simulink library "symbols"  (Simulink 7.5)
settings: Solver=ode45  StartTime=0.0  StopTime=10.0  RelTol=1e-3
libraries: xbsIndex_r4 x41
settings Model: Creator=ich  LastModifiedBy=ich

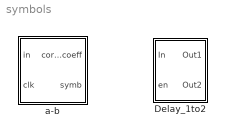
== system symbols ==
  Delay_1to2 : Subsystem
      mask Display:
      | disp('z^{-1}','texmode','on')
      | port_label('input',1,'in')
      | port_label('input',2,'en')
      | port_label('output',1,'out')
      | port_label('output',2,'out')
  a-b : Subsystem  mask{a=0, b=8, chip_a=1618456172}
      mask prompts: a "Symbol a"; b "Symbol b"; chip_a "Chipping seq. for a"

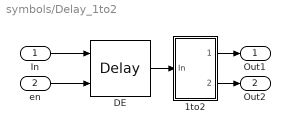
== system symbols/Delay_1to2 ==
  In : Inport
  en : Inport  Port=2
  1to2 : Subsystem
  DE : xbsIndex_r4/Delay  en=on  latency=1  dbl_ovrd=off  reg_retiming=off  block_type=delay
      settings: xl_area=[1 1 0 0 0 0 0]  block_version=12.1
  Out1 : Outport
  Out2 : Outport  Port=2
  wires:
  DE/1 -> 1to2/1(In)
  In/1 -> DE/1
  1to2/1(Out1) -> Out1/1
  1to2/2(Out2) -> Out2/1
  en/1 -> DE/2

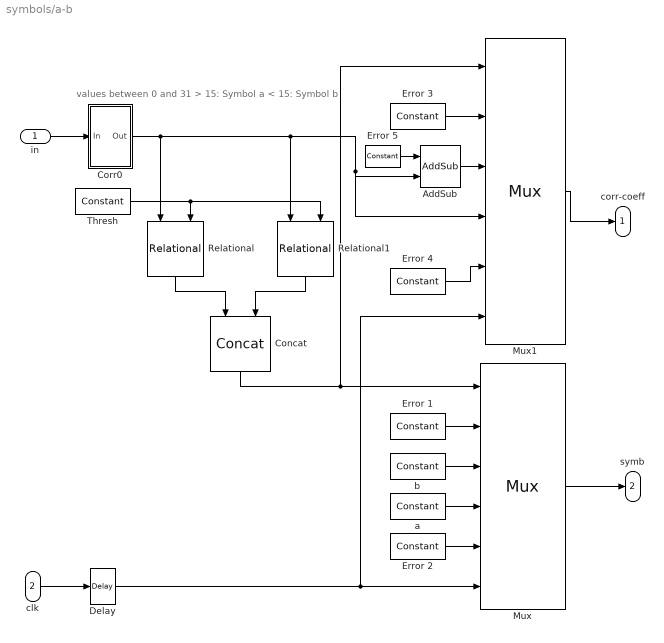
== system symbols/a-b ==
  note: values between 0 and 31
      | > 15: Symbol a
      | < 15: Symbol b
  in : Inport
  clk : Inport  Port=2
  AddSub : xbsIndex_r4/AddSub  mode=Subtraction  use_carryin=off  use_carryout=off  en=off  latency=0  precision=Full  arith_type=Unsigned  n_bits=16  bin_pt=14  quantization=Truncate  overflow=Wrap  dbl_ovrd=off  use_behavioral_HDL=off  hw_selection=Fabric  pipelined=off  block_type=addsub
      settings: block_version=12.2
  Concat : xbsIndex_r4/Concat  num_inputs=2  dbl_ovrd=off  block_type=concat
      settings: block_version=12.1
  Corr0 : Subsystem
  Delay : xbsIndex_r4/Delay  en=off  latency=1  dbl_ovrd=off  reg_retiming=off  block_type=delay
      settings: block_version=12.2
  Error 1 : xbsIndex_r4/Constant  arith_type=Unsigned  const=16  n_bits=5  bin_pt=0  explicit_period=off  period=1  equ=P=C  opselect=C  inp2=PCIN>>17  opr=+  inp1=P  carry=CIN  dbl_ovrd=off  block_type=constant
      settings: block_version=12.1
  Error 2 : xbsIndex_r4/Constant  arith_type=Unsigned  const=16  n_bits=5  bin_pt=0  explicit_period=off  period=1  equ=P=C  opselect=C  inp2=PCIN>>17  opr=+  inp1=P  carry=CIN  dbl_ovrd=off  block_type=constant
      settings: block_version=12.1
  Error 3 : xbsIndex_r4/Constant  arith_type=Unsigned  const=0  n_bits=5  bin_pt=0  explicit_period=off  period=1  equ=P=C  opselect=C  inp2=PCIN>>17  opr=+  inp1=P  carry=CIN  dbl_ovrd=off  block_type=constant
      settings: block_version=12.1
  Error 4 : xbsIndex_r4/Constant  arith_type=Unsigned  const=0  n_bits=5  bin_pt=0  explicit_period=off  period=1  equ=P=C  opselect=C  inp2=PCIN>>17  opr=+  inp1=P  carry=CIN  dbl_ovrd=off  block_type=constant
      settings: block_version=12.1
  Error 5 : xbsIndex_r4/Constant  arith_type=Unsigned  const=31  n_bits=5  bin_pt=0  explicit_period=off  period=1  equ=P=C  opselect=C  inp2=PCIN>>17  opr=+  inp1=P  carry=CIN  dbl_ovrd=off  block_type=constant
      settings: block_version=12.1
  Mux : xbsIndex_r4/Mux  inputs=4  en=on  latency=1  precision=Full  arith_type=Unsigned  n_bits=16  bin_pt=14  quantization=Truncate  overflow=Wrap  dbl_ovrd=off  block_type=mux
      settings: xl_area=[5 5 0 10 0 0 0]  block_version=12.1
  Mux1 : xbsIndex_r4/Mux  inputs=4  en=on  latency=1  precision=Full  arith_type=Unsigned  n_bits=16  bin_pt=14  quantization=Truncate  overflow=Wrap  dbl_ovrd=off  block_type=mux
      settings: xl_area=[5 5 0 10 0 0 0]  block_version=12.1
  Relational : xbsIndex_r4/Relational  mode=a>b  en=off  latency=0  dbl_ovrd=off  block_type=relational
      settings: xl_area=[4 1 0 7 0 0 0]  block_version=12.1
  Relational1 : xbsIndex_r4/Relational  mode=a<=b  en=off  latency=0  dbl_ovrd=off  block_type=relational
      settings: xl_area=[4 1 0 7 0 0 0]  block_version=12.1
  Thresh : xbsIndex_r4/Constant  arith_type=Unsigned  const=15  n_bits=5  bin_pt=0  explicit_period=off  period=1  equ=P=C  opselect=C  inp2=PCIN>>17  opr=+  inp1=P  carry=CIN  dbl_ovrd=off  block_type=constant
      settings: block_version=12.1
  a : xbsIndex_r4/Constant  arith_type=Unsigned  const=a  n_bits=5  bin_pt=0  explicit_period=off  period=1  equ=P=C  opselect=C  inp2=PCIN>>17  opr=+  inp1=P  carry=CIN  dbl_ovrd=off  block_type=constant
      settings: block_version=12.1
  b : xbsIndex_r4/Constant  arith_type=Unsigned  const=b  n_bits=5  bin_pt=0  explicit_period=off  period=1  equ=P=C  opselect=C  inp2=PCIN>>17  opr=+  inp1=P  carry=CIN  dbl_ovrd=off  block_type=constant
      settings: block_version=12.1
  corr-coeff : Outport
  symb : Outport  Port=2
  wires:
  Corr0/1(Out) -> Relational/1, Relational1/1, Mux1/4, AddSub/2
  Thresh/1 -> Relational/2, Relational1/2
  in/1 -> Corr0/1(In)
  Relational/1 -> Concat/1
  Relational1/1 -> Concat/2
  Error 1/1 -> Mux/2
  b/1 -> Mux/3
  a/1 -> Mux/4
  Error 2/1 -> Mux/5
  clk/1 -> Delay/1
  Concat/1 -> Mux/1, Mux1/1
  Mux/1 -> symb/1
  Error 3/1 -> Mux1/2
  Error 4/1 -> Mux1/5
  Mux1/1 -> corr-coeff/1
  AddSub/1 -> Mux1/3
  Error 5/1 -> AddSub/1
  Delay/1 -> Mux/6, Mux1/6

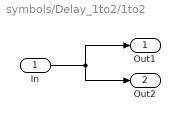
== system symbols/Delay_1to2/1to2 ==
  In : Inport  OutDataType=fixdt(1, 16)  OutScaling=2^0
  Out1 : Outport  OutDataType=fixdt(1, 16)  OutScaling=2^0
  Out2 : Outport  Port=2  OutDataType=fixdt(1, 16)  OutScaling=2^0
  wires:
  In/1 -> Out1/1, Out2/1

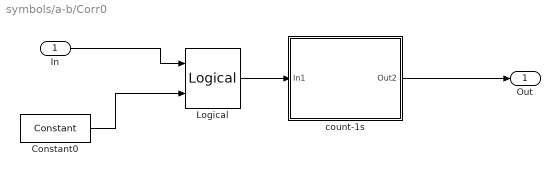
== system symbols/a-b/Corr0 ==
  In : Inport
  Constant0 : xbsIndex_r4/Constant  arith_type=Unsigned  const=chip_a  n_bits=31  bin_pt=0  explicit_period=off  period=1/8  equ=P=C  opselect=C  inp2=PCIN>>17  opr=+  inp1=P  carry=CIN  dbl_ovrd=off  block_type=constant
      settings: block_version=12.1
  Logical : xbsIndex_r4/Logical  logical_function=XNOR  inputs=2  en=off  latency=0  precision=User Defined  arith_type=Unsigned  n_bits=32  bin_pt=0  align_bp=on  dbl_ovrd=off  block_type=logical
      settings: xl_area=[31 0 0 31 0 0 0]  block_version=12.1
  count-1s : Subsystem
  Out : Outport
  wires:
  Constant0/1 -> Logical/2
  Logical/1 -> count-1s/1(In1)
  In/1 -> Logical/1
  count-1s/1(Out2) -> Out/1

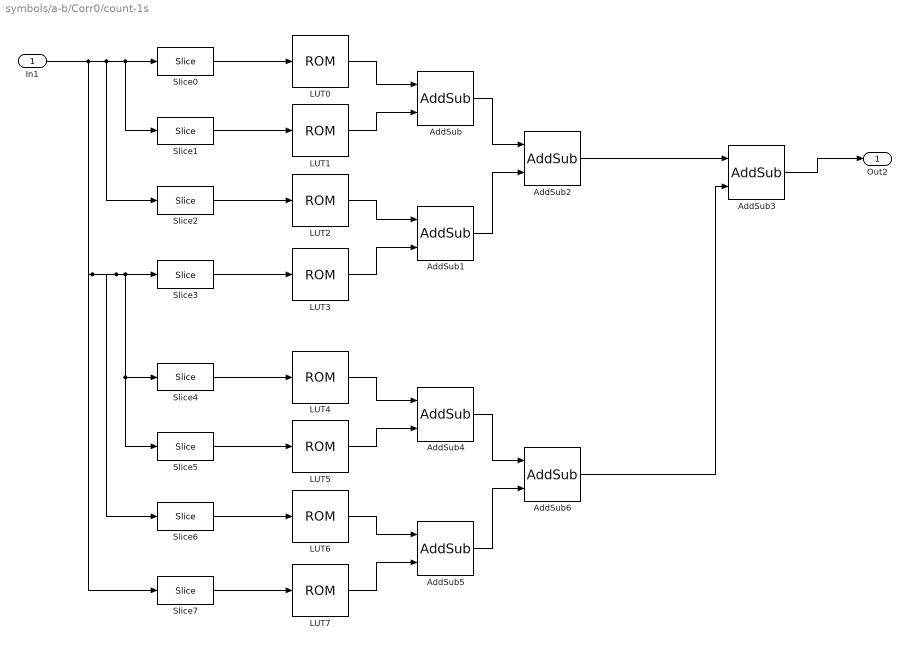
== system symbols/a-b/Corr0/count-1s ==
  In1 : Inport
  AddSub{,1,4..5} (4 alike) : xbsIndex_r4/AddSub  mode=Addition  use_carryin=off  use_carryout=off  en=off  latency=1  precision=Full  arith_type=Unsigned  n_bits=16  bin_pt=14  quantization=Truncate  overflow=Wrap  dbl_ovrd=off  use_behavioral_HDL=off  hw_selection=Fabric  pipelined=off  block_type=addsub
      settings: xl_area=[2 0 0 3 0 0 0]  block_version=12.1
  AddSub2 : xbsIndex_r4/AddSub  mode=Addition  use_carryin=off  use_carryout=off  en=off  latency=0  precision=Full  arith_type=Unsigned  n_bits=16  bin_pt=14  quantization=Truncate  overflow=Wrap  dbl_ovrd=off  use_behavioral_HDL=off  hw_selection=Fabric  pipelined=off  block_type=addsub
      settings: xl_area=[3 0 0 4 0 0 0]  block_version=12.1
  AddSub3 : xbsIndex_r4/AddSub  mode=Addition  use_carryin=off  use_carryout=off  en=off  latency=0  precision=Full  arith_type=Unsigned  n_bits=16  bin_pt=14  quantization=Truncate  overflow=Wrap  dbl_ovrd=off  use_behavioral_HDL=off  hw_selection=Fabric  pipelined=off  block_type=addsub
      settings: xl_area=[3 0 0 5 0 0 0]  block_version=12.1
  AddSub6 : xbsIndex_r4/AddSub  mode=Addition  use_carryin=off  use_carryout=off  en=off  latency=0  precision=Full  arith_type=Unsigned  n_bits=16  bin_pt=14  quantization=Truncate  overflow=Wrap  dbl_ovrd=off  use_behavioral_HDL=off  hw_selection=Fabric  pipelined=off  block_type=addsub
      settings: xl_area=[3 0 0 4 0 0 0]  block_version=12.1
  LUT{0..7} (8 alike) : xbsIndex_r4/ROM  depth=16  initVector=[0,1,1,2,1,2,2,3,1,2,2,3,2,3,3,4]  distributed_mem=Distributed memory  rst=off  init_reg=0  en=off  latency=0  arith_type=Unsigned  n_bits=3  bin_pt=0  dbl_ovrd=off  optimize=Area  use_rpm=on  block_type=sprom
      settings: xl_area=[0 0 1 0 0 0 0]  block_version=12.1
  Slice0 : xbsIndex_r4/Slice  nbits=4  boolean_output=off  mode=Lower Bit Location + Width  bit1=0  base1=MSB of Input  bit0=0  base0=LSB of Input  dbl_ovrd=off  block_type=slice
      settings: block_version=12.1
  Slice1 : xbsIndex_r4/Slice  nbits=4  boolean_output=off  mode=Lower Bit Location + Width  bit1=-4  base1=MSB of Input  bit0=4  base0=LSB of Input  dbl_ovrd=off  block_type=slice
      settings: block_version=12.1
  Slice2 : xbsIndex_r4/Slice  nbits=4  boolean_output=off  mode=Lower Bit Location + Width  bit1=-8  base1=MSB of Input  bit0=8  base0=LSB of Input  dbl_ovrd=off  block_type=slice
      settings: block_version=12.1
  Slice3 : xbsIndex_r4/Slice  nbits=4  boolean_output=off  mode=Lower Bit Location + Width  bit1=-12  base1=MSB of Input  bit0=12  base0=LSB of Input  dbl_ovrd=off  block_type=slice
      settings: block_version=12.1
  Slice4 : xbsIndex_r4/Slice  nbits=4  boolean_output=off  mode=Lower Bit Location + Width  bit1=0  base1=LSB of Input  bit0=16  base0=LSB of Input  dbl_ovrd=off  block_type=slice
      settings: block_version=12.1
  Slice5 : xbsIndex_r4/Slice  nbits=4  boolean_output=off  mode=Lower Bit Location + Width  bit1=0  base1=LSB of Input  bit0=20  base0=LSB of Input  dbl_ovrd=off  block_type=slice
      settings: block_version=12.1
  Slice6 : xbsIndex_r4/Slice  nbits=4  boolean_output=off  mode=Lower Bit Location + Width  bit1=0  base1=LSB of Input  bit0=24  base0=LSB of Input  dbl_ovrd=off  block_type=slice
      settings: block_version=12.1
  Slice7 : xbsIndex_r4/Slice  nbits=4  boolean_output=off  mode=Lower Bit Location + Width  bit1=0  base1=LSB of Input  bit0=28  base0=LSB of Input  dbl_ovrd=off  block_type=slice
      settings: block_version=12.1
  Out2 : Outport
  wires:
  In1/1 -> Slice0/1, Slice1/1, Slice2/1, Slice7/1, Slice6/1, Slice3/1, Slice4/1, Slice5/1
  Slice0/1 -> LUT0/1
  Slice3/1 -> LUT3/1
  Slice2/1 -> LUT2/1
  Slice1/1 -> LUT1/1
  LUT0/1 -> AddSub/1
  LUT1/1 -> AddSub/2
  LUT2/1 -> AddSub1/1
  LUT3/1 -> AddSub1/2
  AddSub1/1 -> AddSub2/2
  AddSub/1 -> AddSub2/1
  AddSub3/1 -> Out2/1
  Slice4/1 -> LUT4/1
  Slice7/1 -> LUT7/1
  Slice6/1 -> LUT6/1
  Slice5/1 -> LUT5/1
  LUT4/1 -> AddSub4/1
  LUT5/1 -> AddSub4/2
  LUT6/1 -> AddSub5/1
  LUT7/1 -> AddSub5/2
  AddSub5/1 -> AddSub6/2
  AddSub4/1 -> AddSub6/1
  AddSub2/1 -> AddSub3/1
  AddSub6/1 -> AddSub3/2
